simulink model "aula10_R2019"  (R2019a)
settings: Solver=FixedStepAuto  StartTime=0.0  StopTime=5  RelTol=1e-3
values from neighbouring files (symbols this model uses):
  u0 = ones(size(u0));u0(1:5)=0    [desempenho.m]
  y0 = y0-y0(1)    [desempenho.m]
undefined symbols (not defined in the file or in its folder): A, B, C, g2, K, Ki, Kp, L, p1, Ref, RI, Ts
libraries: simulink x1
settings Model: Creator=celsojosemunaro  LastModifiedBy=celsojosemunaro

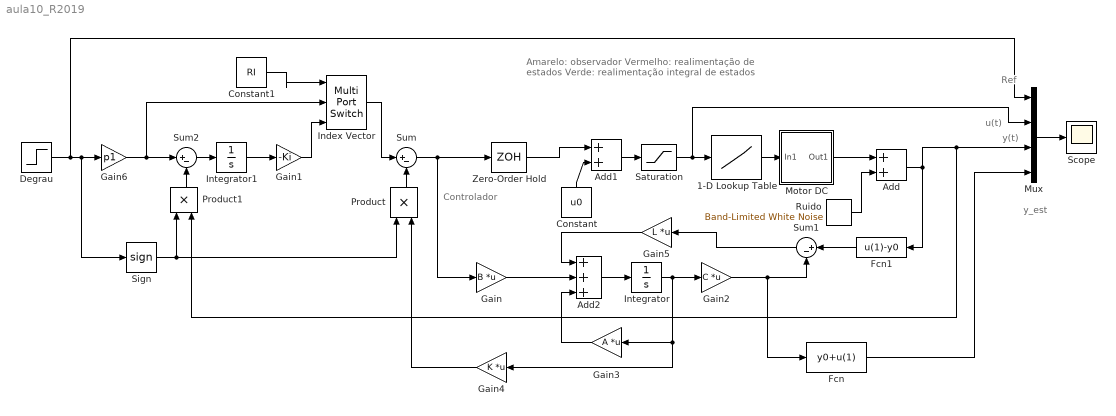
== system aula10_R2019 ==
  note: Amarelo: observador
      | Vermelho: realimentação de estados
      | Verde: realimentação integral de estados
  note: y_est
  note: Controlador
  note: y(t)
  note: u(t)
  note: Ref
  1-D Lookup Table : Lookup_n-D  NumberOfTableDimensions=1  BreakpointsForDimension1=[0,35,37,52,71,91,113,142,164,190,225]  Table=[0,0,330,850,1450,1930,2396,2793,3015,3224,3434]  InternalRulePriority=Speed  RndMeth=Simplest  InputSameDT=on
  Add : Sum
  Add1 : Sum
  Add2 : Sum  Inputs=+++
  Constant : Constant  Value=u0
  Constant1 : Constant  Value=RI
  Degrau : Step  Time=2  After=Ref  SampleTime=Ts
  Fcn : Fcn  Expr=y0+u(1)
  Fcn1 : Fcn  Expr=u(1)-y0
  Gain : Gain  Gain=B  Multiplication=Matrix(K*u)
  Gain1 : Gain  Gain=-Ki
  Gain2 : Gain  Gain=C  Multiplication=Matrix(K*u)
  Gain3 : Gain  Gain=A  Multiplication=Matrix(K*u)
  Gain4 : Gain  Gain=K  Multiplication=Matrix(K*u)
  Gain5 : Gain  Gain=L  Multiplication=Matrix(K*u)
  Gain6 : Gain  Gain=p1
  Index Vector : MultiPortSwitch  DataPortOrder=Zero-based contiguous  Inputs=2  zeroidx=on
  Integrator : Integrator
  Integrator1 : Integrator
  "Motor DC " : Subsystem
  Mux : Mux
  Product : Product
  Product1 : Product
  Ruido : simulink/Sources/Band-Limited White Noise  Cov=0.1  Ts=Ts  seed=[23341]
  Saturation : Saturate  UpperLimit=256  LowerLimit=0
  Scope : Scope
  Sign : Signum
  Sum : Sum  Inputs=|+-
  Sum1 : Sum  Inputs=|+-
  Sum2 : Sum  Inputs=|+-
  Zero-Order Hold : ZeroOrderHold  SampleTime=Ts
  wires:
  Mux/1 -> Scope/1
  "Motor DC "/1(Out1) -> Add/1
  Ruido/1 -> Add/2
  Product/1 -> Sum/2
  Sign/1 -> Product/1, Product1/1
  Constant/1 -> Add1/2
  1-D Lookup Table/1 -> "Motor DC "/1(In1)
  Add1/1 -> Saturation/1
  Saturation/1 -> Mux/2, 1-D Lookup Table/1
  Zero-Order Hold/1 -> Add1/1
  Sum/1 -> Gain/1, Zero-Order Hold/1
  Gain/1 -> Add2/2
  Add2/1 -> Integrator/1
  Integrator/1 -> Gain4/1, Gain3/1, Gain2/1
  Gain3/1 -> Add2/3
  Gain4/1 -> Product/2
  Sum1/1 -> Gain5/1
  Gain5/1 -> Add2/1
  Gain2/1 -> Fcn/1, Sum1/2
  Fcn1/1 -> Sum1/1
  Fcn/1 -> Mux/4
  Degrau/1 -> Mux/1, Sign/1, Gain6/1
  Sum2/1 -> Integrator1/1
  Integrator1/1 -> Gain1/1
  Product1/1 -> Sum2/2
  Add/1 -> Fcn1/1, Product1/2, Mux/3
  Constant1/1 -> Index Vector/1
  Gain1/1 -> Index Vector/3
  Index Vector/1 -> Sum/1
  Gain6/1 -> Index Vector/2, Sum2/1

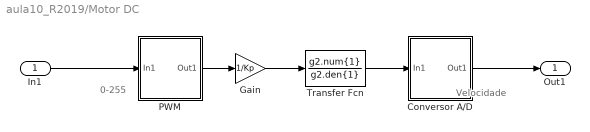
== system aula10_R2019/Motor DC  ==
  note: 0-255
  note: Velocidade
  In1 : Inport
  Conversor A/D : Subsystem
  Gain : Gain  Gain=1/Kp
  PWM : Subsystem
  Transfer Fcn : TransferFcn  Numerator=g2.num{1}  Denominator=g2.den{1}
  Out1 : Outport
  wires:
  Conversor A/D/1(Out1) -> Out1/1
  Transfer Fcn/1 -> Conversor A/D/1(In1)
  PWM/1(Out1) -> Gain/1
  In1/1 -> PWM/1(In1)
  Gain/1 -> Transfer Fcn/1

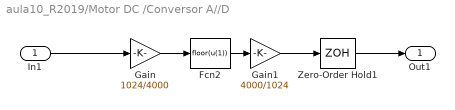
== system aula10_R2019/Motor DC /Conversor A//D ==
  In1 : Inport
  Fcn2 : Fcn  Expr=floor(u(1))
  Gain : Gain  Gain=1024/4000
  Gain1 : Gain  Gain=4000/1024
  Zero-Order Hold1 : ZeroOrderHold  SampleTime=Ts
  Out1 : Outport
  wires:
  Fcn2/1 -> Gain1/1
  Gain/1 -> Fcn2/1
  In1/1 -> Gain/1
  Zero-Order Hold1/1 -> Out1/1
  Gain1/1 -> Zero-Order Hold1/1

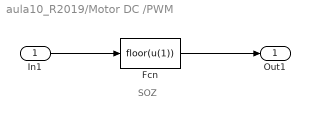
== system aula10_R2019/Motor DC /PWM ==
  note: SOZ
  In1 : Inport
  Fcn : Fcn  Expr=floor(u(1))
  Out1 : Outport
  wires:
  Fcn/1 -> Out1/1
  In1/1 -> Fcn/1
